simulink library "vmc"  (R2021b)
settings: Solver=VariableStepAuto  StartTime=0.0  StopTime=10.0  RelTol=1e-3
undefined symbols (not defined in the file or in its folder): AVMC_ACCDeltaTqIGain_X_kph, AVMC_ACCDeltaTqIGain_Y_mps2, AVMC_ACCDeltaTqPGain_X_kph, AVMC_ACCDeltaTqPGain_Y_kph, AVMC_ACCLongSteadyCtrl_X_kph, AVMC_AggressJerkPCT4AT_X_kph, AVMC_AggressJerkPCT_X_kph, AVMC_AggressLimitPCT4AT_X_kph, AVMC_AggressLimitPCT_X_kph, AVMC_CCLongSteadyCtrl_X_kph, AVMC_DISCDeltaTqIGain_X_kph, AVMC_DISCDeltaTqIGain_Y_mps2, AVMC_DISCDeltaTqPGain_X_kph, AVMC_DISCDeltaTqPGain_Y_kph, AVMC_DISCTrunAccJerk_X_s, AVMC_DISCTrunAccLimit_X_s, AVMC_ESCRegenOut_X_kph, AVMC_ESCRegenOut_Y_Deg, AVMC_ESCRegenOutEnSpd_X_Deg, AVMC_ISOAccLimit_X_mps, AVMC_ISODecLimit_X_mps, AVMC_ISOJerk_X_mps, AVMC_LatESCRegenOut_X_kph, AVMC_LatESCRegenOut_Y_Deg, AVMC_LongAccDeadZone_X_kph, AVMC_LongAccFiltTsforP2_X_Gps, AVMC_MCPresBaseTq_X_bar, AVMC_MSALongSteadyCtrl_X_kph, AVMC_MSAPedalOvrd2_X_kph, AVMC_MSAPedalOvrd_X_kph, AVMC_MSASpdBand_X_kph, AVMC_MSATqDownEndTq_X_kph, AVMC_MSATqDownTime_X_kph, AVMC_RDCDetectTime_X_kph, AVMC_RDCDetectTime_Y_pct, AVMC_RDCEnSlideRate_X_Deg, AVMC_RearWhlTqRatio_X_Nm, AVMC_RearWhlTqRatio_Y_gps, AVMC_RearWhlTqSlipGain_X_rat, AVMC_RearWhlTqSlipGain_Y_kph, AVMC_SoftJerkPCT_X_kph, AVMC_SoftLimitPCT_X_kph, AVMC_StESCYaw_X_kph, AVMC_StESCYaw_Y_Deg, AVMC_StESCYawCom_X_kph, AVMC_StESCYawCom_Y_Gps, AVMC_TMSpdBaseTq_X_rpm, AVMC_VehHoldBDecMap_X_kph, AVMC_VehHoldDecCtrlTime_X_kph, AVMC_VehHoldMCPPass_X_deg, C_TASK_10MS_S, C_TASK_5MS_S, DEG2RAD, Discrete, ENUM_ACCAVAIL_AVAILABLE, ENUM_ACCCTRLALLOW_ALLOW, ENUM_ADASACCSTA_ACTIVE, ENUM_ADASACCSTA_OVERRIDE, ENUM_ADASACCSTA_SHUTOFF, ENUM_ADASAEBREQ_NOREQUEST ... (+361)
libraries: hcu_lib x63, simulink x60, simulink_extras x3, ctrlSharedLib x3, $bdroot x2
(part 9 of 15)

== system vmc/VMC/VMC/RDC Determination/RWD ==
  task_time_s : Inport
  VVMC_ActMaxSlideRate_pct : Inport  Port=2
  VTQD_AfterAvailableTqDemFr_Nm : Inport  Port=3
  VTQD_AfterAvailableTqDemRr_Nm : Inport  Port=4
  VINP_ESCActive_flg : Inport  Port=5
  VINP_SASAngle_Deg : Inport  Port=6
  VINP_LatAccel_Gps : Inport  Port=7
  VINP_VehSpeed_kph : Inport  Port=8
  VINP_YawRate_degps : Inport  Port=9
  VINP_RDCActive_enum : Inport  Port=10
  VINP_DIDGetDynoMode_flg : Inport  Port=11
  AND{,2..5} (5 alike) : Logic  AllPortsSameDT=off  OutDataTypeStr=boolean
  AND1 : Logic  Inputs=3  AllPortsSameDT=off  OutDataTypeStr=boolean
  Abs{,1..7} (8 alike) : Abs
  Add1 : Sum
  Constant1 : Constant  Value=ZERO_INT
  Constant2 : Constant  Value=KVMC_DIDGetDynoModeSW_flg
  Constant{3..4,74,78} (4 alike) : Constant  Value=KVMC_AltRDCActiveTq_Nm
  Constant73 : Constant  Value=ENUM_RDCACTSTA_NOREQUEST
  Constant77 : Constant  Value=ENUM_RDCACTSTA_RAMPOUT
  Constant81 : Constant  Value=KVMC_AltRDCActiveSW_flg
  Constant82 : Constant  Value=ENUM_RDCACTSTA_EXITIMMEDIATELY
  Constant83 : Constant  Value=KVMC_AltRDCRecTime_s
  Constant86 : Constant  Value=KVMC_ESCRegenTqRecDelay_s
  Constant95 : Constant  Value=ENUM_RDCACTSTA_EXITIMMEDIATELY
  Delay{1..2,6..7} (4 alike) : Delay  DelayLength=1
  DelayEnable1 : hcu_lib/Basic_Blocks/DelayEnable
  DelayEnable2 : hcu_lib/Basic_Blocks/DelayEnable
  DelayEnable3 : hcu_lib/Basic_Blocks/DelayEnable
  Equal33 : RelationalOperator  Operator===  OutDataTypeStr=boolean  RndMeth=Simplest
  MVMC_ESCRegenOutEnSpd_Y_kph : Lookup_n-D  NumberOfTableDimensions=1  BreakpointsForDimension1=AVMC_ESCRegenOutEnSpd_X_Deg  Table=MVMC_ESCRegenOutEnSpd_Y_kph  ExtrapMethod=Clip  InternalRulePriority=Speed  RndMeth=Simplest  InputSameDT=on
  MVMC_ESCRegenOut_Z_Dps : Lookup_n-D  BreakpointsForDimension1=AVMC_ESCRegenOut_Y_Deg  BreakpointsForDimension2=AVMC_ESCRegenOut_X_kph  Table=MVMC_ESCRegenOut_Z_Dps  ExtrapMethod=Clip  InternalRulePriority=Speed  RndMeth=Simplest  InputSameDT=on
      settings: InputPortMap=u0,u1
  MVMC_LatESCRegenOut_Z_Gps : Lookup_n-D  BreakpointsForDimension1=AVMC_LatESCRegenOut_Y_Deg  BreakpointsForDimension2=AVMC_LatESCRegenOut_X_kph  Table=MVMC_LatESCRegenOut_Z_Gps  ExtrapMethod=Clip  InternalRulePriority=Speed  RndMeth=Simplest  InputSameDT=on
      settings: InputPortMap=u0,u1
  MVMC_RDCDetectTime_Z_s : Lookup_n-D  BreakpointsForDimension1=AVMC_RDCDetectTime_Y_pct  BreakpointsForDimension2=AVMC_RDCDetectTime_X_kph  Table=MVMC_RDCDetectTime_Z_s  ExtrapMethod=Clip  InternalRulePriority=Speed  RndMeth=Simplest  InputSameDT=on
      settings: InputPortMap=u0,u1
  MVMC_RDCEnSlideRate_Y_pct : Lookup_n-D  NumberOfTableDimensions=1  BreakpointsForDimension1=AVMC_RDCEnSlideRate_X_Deg  Table=MVMC_RDCEnSlideRate_Y_pct  ExtrapMethod=Clip  InternalRulePriority=Speed  RndMeth=Simplest  InputSameDT=on
  MVMC_StESCYawCom_Z_Dps : Lookup_n-D  BreakpointsForDimension1=AVMC_StESCYawCom_Y_Gps  BreakpointsForDimension2=AVMC_StESCYawCom_X_kph  Table=MVMC_StESCYawCom_Z_Dps  ExtrapMethod=Clip  InternalRulePriority=Speed  RndMeth=Simplest  InputSameDT=on
      settings: InputPortMap=u0,u1
  MVMC_StESCYaw_Z_Dps : Lookup_n-D  BreakpointsForDimension1=AVMC_StESCYaw_Y_Deg  BreakpointsForDimension2=AVMC_StESCYaw_X_kph  Table=MVMC_StESCYaw_Z_Dps  ExtrapMethod=Clip  InternalRulePriority=Speed  RndMeth=Simplest  InputSameDT=on
      settings: InputPortMap=u0,u1
  NOT : Logic  Operator=NOT  AllPortsSameDT=off  OutDataTypeStr=boolean
  NOT1 : Logic  Operator=NOT  AllPortsSameDT=off  OutDataTypeStr=boolean
  NOT3 : Logic  Operator=NOT  AllPortsSameDT=off  OutDataTypeStr=boolean
  OR{,1..2,4,9} (5 alike) : Logic  Operator=OR  AllPortsSameDT=off  OutDataTypeStr=boolean
  OR8 : Logic  AllPortsSameDT=off  OutDataTypeStr=boolean
  Relational Operator{1,8..10} (4 alike) : RelationalOperator  OutDataTypeStr=boolean  RndMeth=Simplest
  Relational Operator{2..7} (6 alike) : RelationalOperator  Operator=<=  OutDataTypeStr=boolean  RndMeth=Simplest
  SR_Latch4 : hcu_lib/Basic_Blocks/SR_Latch
  SR_Latch5 : hcu_lib/Basic_Blocks/SR_Latch
  Switch10 : Switch  Criteria=u2 > Threshold
  Switch11 : Switch  Criteria=u2 > Threshold
  Switch8 : Switch  Criteria=u2 > Threshold
  VVMC_RWDRDCActive_enum : Outport
  VVMC_RDCEnSlideRate_pct : Outport  Port=2
  VVMC_ActStESCYaw_Dps : Outport  Port=3
  wires:
  [VVMC_RDCDetectTime_s] -> DelayEnable1/2
  MVMC_RDCEnSlideRate_Y_pct/1 -> VVMC_RDCEnSlideRate_pct/1, [VVMC_RDCEnSlideRate_pct]  "VVMC_RDCEnSlideRate_pct"
  VINP_YawRate_degps/1 -> [VINP_YawRate_degps]
  [VINP_ESCActive_flg] -> NOT1/1
  VINP_ESCActive_flg/1 -> [VINP_ESCActive_flg]
  OR2/1 -> AND3/1
  Constant73/1 -> Switch8/3
  Delay7/1 -> Relational Operator3/1
  VINP_LatAccel_Gps/1 -> [VINP_LatAccel_Gps]
  [VVMC_RDCEnSlideRate_pct] -> Relational Operator1/2
  Switch11/1 -> [VVMC_AltRDCActive_enum]  "VVMC_AltRDCActive_enum"
  VINP_VehSpeed_kph/1 -> [VINP_VehSpeed_kph]
  Constant78/1 -> Relational Operator3/2
  [VINP_SASAngle_Deg] -> Abs7/1
  VVMC_ActMaxSlideRate_pct/1 -> [VVMC_ActMaxSlideRate_pct]
  DelayEnable2/1 -> SR_Latch4/2  "VVMC_AltRDCRec_flg"
  [task_time_s] -> DelayEnable1/3
  OR9/1 -> AND4/1
  [VINP_SASAngle_Deg] -> MVMC_LatESCRegenOut_Z_Gps/1
  [VVMC_ActMaxSlideRate_pct] -> MVMC_RDCDetectTime_Z_s/1
  [VINP_LatAccel_Gps] -> Abs5/1
  VTQD_AfterAvailableTqDemRr_Nm/1 -> [VTQD_AfterAvailableTqDemRr_Nm]
  SR_Latch5/1 -> [VVMC_ESCActive_flg]  "VVMC_ESCActive_flg"
  Abs4/1 -> Relational Operator8/1
  DelayEnable1/1 -> SR_Latch4/1  "VVMC_RDCDetectEn_flg"
  Relational Operator8/1 -> OR9/2
  Constant74/1 -> Relational Operator2/2
  [VVMC_ESCSlip_flg] -> SR_Latch5/1
  Abs5/1 -> Relational Operator10/1
  [VINP_SASAngle_Deg] -> MVMC_ESCRegenOut_Z_Dps/1
  [VINP_VehSpeed_kph] -> Relational Operator9/1
  Switch8/1 -> Switch11/3
  NOT3/1 -> OR8/1
  [VTQD_AfterAvailableTqDemFr_Nm] -> Delay6/1
  Delay6/1 -> Relational Operator2/1
  MVMC_RDCDetectTime_Z_s/1 -> [VVMC_RDCDetectTime_s]  "VVMC_RDCDetectTime_s"
  [VTQD_AfterAvailableTqDemRr_Nm] -> Delay7/1
  [VINP_SASAngle_Deg] -> MVMC_RDCEnSlideRate_Y_pct/1
  AND3/1 -> DelayEnable1/1
  [VVMC_ESCActive_flg] -> OR4/1
  Relational Operator3/1 -> OR2/2
  Relational Operator9/1 -> AND4/2, AND1/1
  Relational Operator1/1 -> AND3/2
  MVMC_ESCRegenOut_Z_Dps/1 -> Relational Operator8/2  "VVMC_ESCRegenOut_Dps"
  [VINP_YawRate_degps] -> Abs4/1
  SR_Latch4/1 -> Switch8/2
  [VVMC_ActMaxSlideRate_pct] -> Abs2/1
  Switch10/1 -> VVMC_RWDRDCActive_enum/1  "VVMC_RWDRDCActive_enum"
  [VINP_RDCActive_enum] -> Equal33/1
  VINP_SASAngle_Deg/1 -> [VINP_SASAngle_Deg]
  [task_time_s] -> DelayEnable3/3
  Abs2/1 -> Relational Operator1/1
  MVMC_LatESCRegenOut_Z_Gps/1 -> Relational Operator10/2  "VVMC_LatESCRegenOut_Gps"
  NOT1/1 -> OR8/2
  Equal33/1 -> OR4/2
  [VINP_VehSpeed_kph] -> MVMC_LatESCRegenOut_Z_Gps/2
  [VVMC_ESCSlip_flg] -> NOT3/1
  Relational Operator2/1 -> OR2/1
  Relational Operator10/1 -> OR9/1
  Constant95/1 -> Switch11/1
  [VINP_VehSpeed_kph] -> MVMC_ESCRegenOut_Z_Dps/2
  OR8/1 -> DelayEnable3/1
  OR4/1 -> Switch11/2
  [VVMC_AltRDCActive_enum] -> Switch10/1
  DelayEnable3/1 -> SR_Latch5/2
  Constant77/1 -> Switch8/1
  Constant86/1 -> DelayEnable3/2
  Constant82/1 -> Equal33/2
  VTQD_AfterAvailableTqDemFr_Nm/1 -> [VTQD_AfterAvailableTqDemFr_Nm]
  VINP_RDCActive_enum/1 -> [VINP_RDCActive_enum]
  task_time_s/1 -> [task_time_s]
  Constant1/1 -> Switch10/3
  [VINP_LatAccel_Gps] -> Abs1/1
  [VINP_SASAngle_Deg] -> Abs/1
  Abs/1 -> MVMC_StESCYaw_Z_Dps/1
  Add1/1 -> VVMC_ActStESCYaw_Dps/1, [VVMC_ActStESCYaw_Dps]  "VVMC_ActStESCYaw_Dps"
  MVMC_StESCYaw_Z_Dps/1 -> Add1/1  "VVMC_StESCYaw_Dps"
  [VINP_VehSpeed_kph] -> MVMC_StESCYaw_Z_Dps/2
  [VINP_VehSpeed_kph] -> MVMC_StESCYawCom_Z_Dps/2
  MVMC_StESCYawCom_Z_Dps/1 -> Add1/2  "VVMC_StESCYawCom_Dps"
  Abs1/1 -> MVMC_StESCYawCom_Z_Dps/1
  [VINP_VehSpeed_kph] -> MVMC_RDCDetectTime_Z_s/2
  AND/1 -> DelayEnable2/1
  [task_time_s] -> DelayEnable2/3
  Relational Operator4/1 -> AND/1
  [VVMC_ActStESCYaw_Dps] -> Relational Operator6/2
  [VVMC_RDCEnSlideRate_pct] -> Relational Operator4/2
  Abs6/1 -> Relational Operator6/1
  Relational Operator6/1 -> AND/2
  Abs3/1 -> Relational Operator4/1
  [VVMC_ActMaxSlideRate_pct] -> Abs3/1
  Constant83/1 -> DelayEnable2/2
  [VINP_YawRate_degps] -> Abs6/1
  Abs7/1 -> MVMC_ESCRegenOutEnSpd_Y_kph/1
  MVMC_ESCRegenOutEnSpd_Y_kph/1 -> Relational Operator9/2  "VVMC_ESCRegenOutEnSpd_kph"
  Constant4/1 -> Relational Operator7/2
  Delay1/1 -> Relational Operator5/1
  [VTQD_AfterAvailableTqDemRr_Nm] -> Delay2/1
  Constant3/1 -> Relational Operator5/2
  Delay2/1 -> Relational Operator7/1
  Relational Operator7/1 -> OR1/2
  Relational Operator5/1 -> OR1/1
  [VTQD_AfterAvailableTqDemFr_Nm] -> Delay1/1
  OR1/1 -> AND1/3
  [VINP_ESCActive_flg] -> AND1/2
  AND4/1 -> OR/1
  AND1/1 -> OR/2
  OR/1 -> [VVMC_ESCSlip_flg]  "VVMC_ESCSlip_flg"
  Constant81/1 -> AND2/1
  AND5/1 -> NOT/1
  Constant2/1 -> AND5/2
  [VINP_DIDGetDynoMode_flg] -> AND5/1
  NOT/1 -> AND2/2
  AND2/1 -> Switch10/2
  VINP_DIDGetDynoMode_flg/1 -> [VINP_DIDGetDynoMode_flg]

== system vmc/VMC/VMC/SPD2ACC/ISO22179 ==
  VVMC_MeterSpdCalcu_mps : Inport
  VVMC_LimitPCT_pct : Inport  Port=2
  Constant : Constant  Value=pct
  Constant1 : Constant  Value=MINUSONE_FLOAT
  Divide : Product  Inputs=**
  Divide1 : Product  Inputs=**
  Divide2 : Product  Inputs=*/
  Divide3 : Product  Inputs=**
  MVMC_ISOAccLimit_Y_mps2 : Lookup_n-D  NumberOfTableDimensions=1  BreakpointsForDimension1=AVMC_ISOAccLimit_X_mps  UseOneInputPortForAllInputData=on  Table=MVMC_ISOAccLimit_Y_mps2  UseLastTableValue=on  InternalRulePriority=Speed  RndMeth=Simplest  InputSameDT=on
  MVMC_ISODecLimit_Y_mps2 : Lookup_n-D  NumberOfTableDimensions=1  BreakpointsForDimension1=AVMC_ISODecLimit_X_mps  UseOneInputPortForAllInputData=on  Table=MVMC_ISODecLimit_Y_mps2  UseLastTableValue=on  InternalRulePriority=Speed  RndMeth=Simplest  InputSameDT=on
  MVMC_ISOJerk_Y_mps3 : Lookup_n-D  NumberOfTableDimensions=1  BreakpointsForDimension1=AVMC_ISOJerk_X_mps  UseOneInputPortForAllInputData=on  Table=MVMC_ISOJerk_Y_mps3  UseLastTableValue=on  InternalRulePriority=Speed  RndMeth=Simplest  InputSameDT=on
  VVMC_ISOAccLimit_mps2 : Outport
  VVMC_ISODecLimit_mps2 : Outport  Port=2
  VVMC_ISOJerkLimit_mps3 : Outport  Port=3
  wires:
  Constant1/1 -> Divide3/1
  [VVMC_ISOJerkLimit_mps3] -> VVMC_ISOJerkLimit_mps3/1  "VVMC_ISOJerkLimit_mps3"
  [VVMC_ISODecLimit_mps2] -> VVMC_ISODecLimit_mps2/1  "VVMC_ISODecLimit_mps2"
  [VVMC_ISOAccLimit_mps2] -> VVMC_ISOAccLimit_mps2/1  "VVMC_ISOAccLimit_mps2"
  [VVMC_MeterSpdCalcu_mps] -> MVMC_ISOJerk_Y_mps3/1
  Constant/1 -> Divide2/2
  [VVMC_LimitPCT_pct] -> Divide2/1
  VVMC_LimitPCT_pct/1 -> [VVMC_LimitPCT_pct]
  VVMC_MeterSpdCalcu_mps/1 -> [VVMC_MeterSpdCalcu_mps]
  Divide/1 -> [VVMC_ISOAccLimit_mps2]
  MVMC_ISOJerk_Y_mps3/1 -> [VVMC_ISOJerkLimit_mps3]
  Divide1/1 -> [VVMC_ISODecLimit_mps2]
  MVMC_ISOAccLimit_Y_mps2/1 -> Divide/2
  [VVMC_MeterSpdCalcu_mps] -> MVMC_ISODecLimit_Y_mps2/1
  Divide3/1 -> Divide1/1
  Divide2/1 -> Divide1/2, Divide/1
  MVMC_ISODecLimit_Y_mps2/1 -> Divide3/2
  [VVMC_MeterSpdCalcu_mps] -> MVMC_ISOAccLimit_Y_mps2/1

== system vmc/VMC/VMC/SPD2ACC/PID ==
  VVMC_SPD2ACCAct_flg : Inport
  VVMC_FeatReqSpd_kph : Inport  Port=2
  VINP_VehSpeed_kph : Inport  Port=3
  VVMC_MeterIndSpeedForCalcu_kph : Inport  Port=4
  Cast To Single : DataTypeConversion  OutDataTypeStr=single
  Constant1 : Constant  Value=ZERO_FLOAT
  Constant10 : Constant  Value=ONE_FLOAT
  Constant2 : Constant  Value=KPH2MPS
  Constant3 : Constant  Value=KPH2MPS
  Constant4 : Constant  Value=ZERO_FLOAT
  Constant5 : Constant  Value=KVMC_PParm_enum
  Constant6 : Constant  Value=KVMC_IParm_enum
  Constant7 : Constant  Value=KVMC_CMDCycleTime_s
  Constant8 : Constant  Value=ZERO_FLOAT
  Constant9 : Constant  Value=KVMC_AccelIGain_enum
  Divide{,1..2,4..5} (5 alike) : Product  Inputs=**
  Divide3 : Product  Inputs=*/
  InitialCondition: 0 : UnitDelay  SampleTime=-1  HasFrameUpgradeWarning=on
  Subtract : Sum
  Sum1 : Sum  Inputs=|+-
  Sum2 : Sum  Inputs=|+-
  Sum4 : Sum  Inputs=|++
  u2 > 0 : Switch  Criteria=u2 > Threshold
  u2 > 0 (1) : Switch  Criteria=u2 > Threshold
  u2 > 0 (2) : Switch  Criteria=u2 > Threshold
  u2 >= 0 : Switch
  VVMC_AccCalcuPID_mps2 : Outport
  VVMC_MeterSpdCalcu_mps : Outport  Port=2
  wires:
  Divide4/1 -> [VVMC_MeterSpdCalcu_mps]
  Constant7/1 -> Cast To Single/1
  Cast To Single/1 -> Divide3/2
  Sum4/1 -> Divide1/2
  Constant8/1 -> u2 > 0 (2)/3
  Constant1/1 -> u2 > 0 (1)/3
  [VVMC_MeterIndSpeedForCalcu_kph] -> Sum1/2, Divide4/1
  Divide3/1 -> [VVMC_AccCalcuPID_mps2]
  Divide/1 -> Subtract/2
  u2 > 0 (1)/1 -> Divide/1
  [VVMC_SPD2ACCAct_flg] -> u2 > 0 (1)/2
  Constant5/1 -> Divide/2
  Divide2/1 -> Divide3/1
  Constant3/1 -> Divide4/2
  [VINP_VehSpeed_kph] -> Sum2/2
  Sum1/1 -> u2 > 0 (2)/2, u2 > 0 (1)/1
  Divide1/1 -> Subtract/1
  Subtract/1 -> Divide2/1
  u2 > 0 (2)/1 -> u2 >= 0/1
  [VVMC_SPD2ACCAct_flg] -> u2 > 0/2
  Constant6/1 -> Divide5/2
  Sum2/1 -> u2 > 0/1, u2 >= 0/2
  [VVMC_FeatReqSpd_kph] -> Sum2/1
  u2 > 0/1 -> Sum4/1, InitialCondition: 0/1
  Constant4/1 -> u2 > 0/3
  InitialCondition: 0/1 -> Sum4/2
  Divide5/1 -> Divide1/1
  Constant2/1 -> Divide2/2
  Constant10/1 -> u2 >= 0/3
  Constant9/1 -> u2 > 0 (2)/1
  u2 >= 0/1 -> Divide5/1
  [VVMC_FeatReqSpd_kph] -> Sum1/1
  VINP_VehSpeed_kph/1 -> [VINP_VehSpeed_kph]
  [VVMC_MeterSpdCalcu_mps] -> VVMC_MeterSpdCalcu_mps/1  "VVMC_MeterSpdCalcu_mps"
  [VVMC_AccCalcuPID_mps2] -> VVMC_AccCalcuPID_mps2/1  "VVMC_AccCalcuPID_mps2"
  VVMC_MeterIndSpeedForCalcu_kph/1 -> [VVMC_MeterIndSpeedForCalcu_kph]
  VVMC_FeatReqSpd_kph/1 -> [VVMC_FeatReqSpd_kph]
  VVMC_SPD2ACCAct_flg/1 -> [VVMC_SPD2ACCAct_flg]
